simulink model "ConstructionCradleControl"  (R2023a)
settings: Solver=ode1be  StartTime=0.0  StopTime=10  FixedStep=1e-3  RelTol=1e-3
undefined symbols (not defined in the file): kd, ki, kp, s
settings Model: Creator=Ilya_Andriyanov  LastModifiedBy=ПК

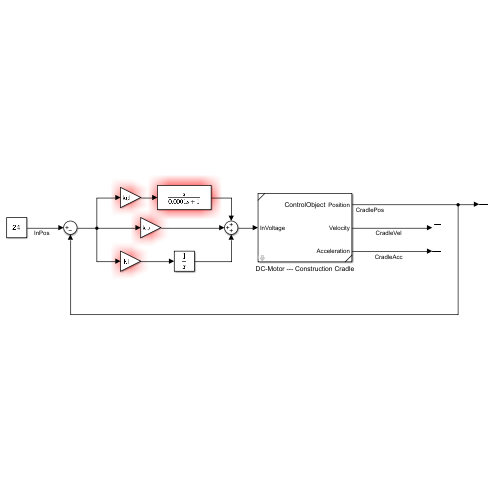
[thumbnail: Simulink's stored preview of the top-level diagram]
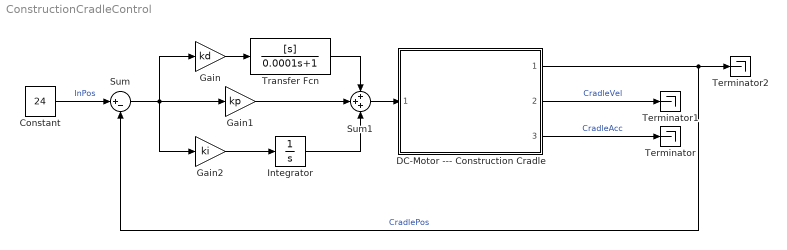
== system ConstructionCradleControl ==
  Constant : Constant  Value=24
  DC-Motor --- Construction Cradle : Subsystem  ReferencedSubsystem=ControlObject  motor_nominal_voltage=24  L=300e-6  R=8.5  km=17e-1  kw=17e-2  J_motor=500e-9  vis_friction_coef_motor=0.001  i_gear=200  J_gear=2.4e-9  vis_friction_coef_gear=0.001  r_cyl=0.3  vis_friction_coef_cradle=0.001  cradle_mass=5
  Gain : Gain  Gain=kd
  Gain1 : Gain  Gain=kp
  Gain2 : Gain  Gain=ki
  Integrator : Integrator
  Sum : Sum  Inputs=|+-
  Sum1 : Sum  Inputs=+++
  Terminator : Terminator
  Terminator1 : Terminator
  Terminator2 : Terminator
  Transfer Fcn : TransferFcn  Numerator=[s]  Denominator=[0.0001 1]
  wires:
  DC-Motor --- Construction Cradle/2 -> Terminator1/1  "CradleVel"
  DC-Motor --- Construction Cradle/3 -> Terminator/1  "CradleAcc"
  Constant/1 -> Sum/1  "InPos"
  Gain/1 -> Transfer Fcn/1
  Sum/1 -> Gain2/1, Gain1/1, Gain/1
  Transfer Fcn/1 -> Sum1/1
  Sum1/1 -> DC-Motor --- Construction Cradle/1
  Gain1/1 -> Sum1/2
  Gain2/1 -> Integrator/1
  Integrator/1 -> Sum1/3
  DC-Motor --- Construction Cradle/1 -> Sum/2, Terminator2/1  "CradlePos"
